simulink model "no_control1"  (R2018a)
settings: Solver=FixedStepAuto  StartTime=0.0  StopTime=50  FixedStep=2e-3  RelTol=1.0e-4
model workspace (MAT data in the model file):
  x1 = Simulink.Parameter
  x1.DataType = 'auto'
  x1.Dimensions = [0 0]
settings Model: Creator=Jay  LastModifiedBy=Jay
settings SolverCC: MaxConsecutiveZCs=1  ExtrapolationOrder=2  InsertRTBMode=Always

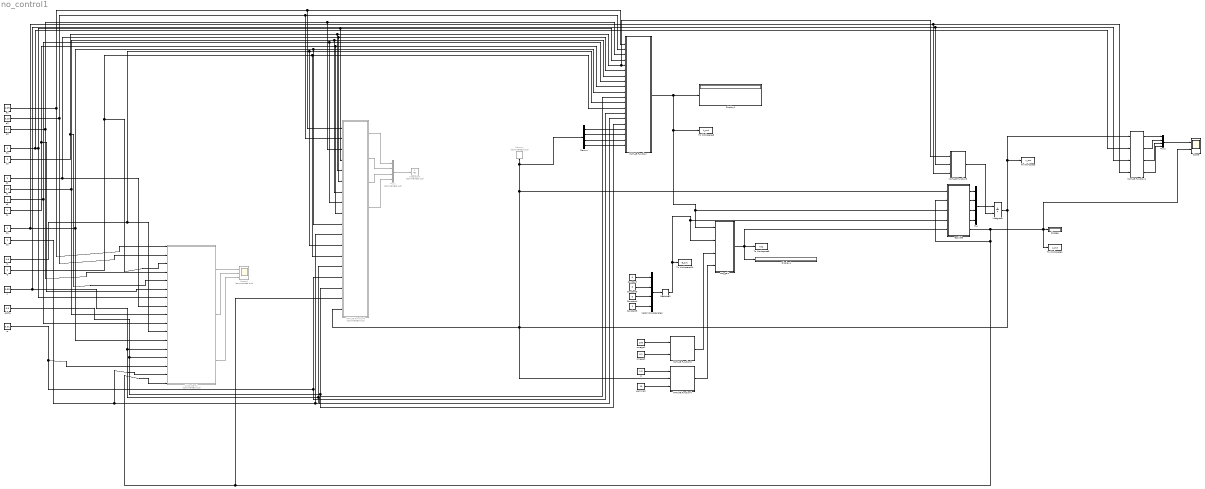
== system no_control1 ==
  Constant : Constant  Value=0
  Constant3 : Constant  Value=0
  Constant4 : Constant  Value=0
  Constant5 : Constant
  Demux : Demux
  Display1 : Display
  Display4 : Display
  Integrator : Integrator  InitialConditionSource=external  InitialCondition=[ 1-1; 0.2; 0.15-0.33/1; 0]
  Integrator2 : Integrator  Commented=on  InitialCondition=[1-1;0.2;0.15-0.33/0.2;0]
  MATLAB Function : MATLAB Function  TreatAsAtomicUnit=on
  MATLAB Function1 : MATLAB Function  TreatAsAtomicUnit=on
  MATLAB Function3 : MATLAB Function  TreatAsAtomicUnit=on
  MATLAB Function4 : MATLAB Function  TreatAsAtomicUnit=on
  MATLAB Function5 : MATLAB Function  TreatAsAtomicUnit=on
  MATLAB Function8 : MATLAB Function  Commented=on  TreatAsAtomicUnit=on
  Memory : Memory  Commented=on  InitialCondition=[0; 0.2; 0.15-0.33/1; 0]  InheritSampleTime=on
  Mux : Mux
  Mux1 : Mux  Commented=on
  Mux2 : Mux
  Reshape2 : Reshape  OutputDimensionality=Column vector (2-D)
  Scope : Scope  NumInputPorts=2
  Scope1 : Scope  Commented=on  NumInputPorts=3
  Subsystem1 : Subsystem  Commented=on
  To Workspace : ToWorkspace  VariableName=x_out  SaveFormat=Timeseries  SampleTime=-1
  To Workspace1 : ToWorkspace  VariableName=u_out  SaveFormat=Timeseries  SampleTime=-1
  To Workspace10 : ToWorkspace  VariableName=B_out  SaveFormat=Timeseries  SampleTime=-1
  To Workspace8 : ToWorkspace  VariableName=A_out  SaveFormat=Timeseries  SampleTime=-1
  To Workspace9 : ToWorkspace  VariableName=Kop  SaveFormat=Timeseries  SampleTime=-1
  Vector Concatenate2 : Concatenate  NumInputs=4  ConcatenateDimension=4
  a1 : Constant  Value=0.05
  a2 : Constant  Value=0.15
  a3 : Constant  Value=0.1
  alpha : Constant  Value=0.3
  are_gain : MATLAB Function  TreatAsAtomicUnit=on
  b1 : Constant
  b2 : Constant
  c1 : Constant
  c2 : Constant  Value=0.5
  c3 : Constant
  c4 : Constant
  d1 : Constant
  d2 : Constant
  dosage : Display
  gamma0 : Constant  Value=10
  omega1 : Constant  Value=100
  omega2 : Constant  Value=0.1
  r1 : Constant  Value=1.5
  r2 : Constant
  rc : Constant  Value=1.2
  regulate : MATLAB Function  TreatAsAtomicUnit=on
  ro : Constant  Value=0.01
  s : Constant  Value=0.33
  wires:
  regulate/5(u) -> regulate/2("u "), Subsystem1/17(u), MATLAB Function8/17(u), To Workspace1/1, dosage/1, Scope/2  "u"
  are_gain/1(Kop) -> regulate/5(Kop), To Workspace9/1, Display4/1
  MATLAB Function4/1(R) -> are_gain/4(R)  "R"
  MATLAB Function3/1(Q) -> are_gain/3(Q)  "Q"
  d2/1 -> Subsystem1/16(d2), MATLAB Function/11(d2), MATLAB Function8/11(d2)  "d2"
  omega1/1 -> MATLAB Function3/1(omega1)
  ro/1 -> MATLAB Function/14(ro), MATLAB Function8/15(ro), Subsystem1/15(ro)  "ro"
  c1/1 -> Subsystem1/8(c1), MATLAB Function8/6(c1), MATLAB Function/6(c1)  "c1"
  Reshape2/1 -> are_gain/2(B), regulate/4(B), To Workspace10/1  "B"
  Constant3/1 -> Vector Concatenate2/2
  gamma0/1 -> MATLAB Function4/3(gamma0)
  b1/1 -> MATLAB Function1/2(b1), Subsystem1/7(b1), MATLAB Function8/4(b1), MATLAB Function/4(b1)  "b1"
  alpha/1 -> MATLAB Function/16(alpha), MATLAB Function8/16(alpha), Subsystem1/14(alpha)  "alpha"
  d1/1 -> MATLAB Function1/4(d1), MATLAB Function5/3(d1), Subsystem1/12(d1), MATLAB Function/10(d1), MATLAB Function8/10(d1)  "d1"
  Constant4/1 -> Vector Concatenate2/3
  r1/1 -> Subsystem1/11(r1), MATLAB Function/12(r1), MATLAB Function8/12(r1)  "r1"
  a2/1 -> Subsystem1/2(a2), MATLAB Function/2(a2), MATLAB Function8/2(a2)  "a2"
  a3/1 -> Subsystem1/4(a3), MATLAB Function/3(a3), MATLAB Function8/3(a3)  "a3"
  c4/1 -> Subsystem1/6(c4), MATLAB Function8/9(c4), MATLAB Function/9(c4)  "c4"
  b2/1 -> Subsystem1/5(b2), MATLAB Function8/5(b2), MATLAB Function/5(b2), MATLAB Function5/1(b2)  "b2"
  Vector Concatenate2/1 -> Reshape2/1
  rc/1 -> MATLAB Function4/1(rc)
  Constant/1 -> Vector Concatenate2/1
  omega2/1 -> MATLAB Function3/2(omega2)
  MATLAB Function/1(A) -> regulate/3(A), are_gain/1(A), To Workspace8/1, Display1/1  "A"
  c2/1 -> Subsystem1/9(c2), MATLAB Function8/7(c2), MATLAB Function/7(c2)  "c2"
  r2/1 -> Subsystem1/3(r2), MATLAB Function/13(r2), MATLAB Function8/13(r2)  "r2"
  c3/1 -> Subsystem1/10(c3), MATLAB Function/8(c3), MATLAB Function8/8(c3)  "c3"
  a1/1 -> Subsystem1/1(a1), MATLAB Function/1(a1), MATLAB Function8/1(a1)  "a1"
  s/1 -> MATLAB Function/15(s), MATLAB Function8/14(s), Subsystem1/13(s), MATLAB Function1/3(s), MATLAB Function5/2(s)  "s"
  Integrator/1 -> MATLAB Function1/1(x), To Workspace/1, MATLAB Function4/2(x), Demux/1, Memory/1, regulate/1(x), MATLAB Function8/18(x)  "x"
  MATLAB Function8/1(x1_dot) -> Mux1/1
  MATLAB Function8/2(x2_dot) -> Mux1/2
  MATLAB Function8/3(x3_dot) -> Mux1/3
  MATLAB Function1/1(N) -> Mux2/1  "N"
  MATLAB Function1/2(T) -> Mux2/2  "T"
  MATLAB Function1/3(I) -> Mux2/3  "I"
  MATLAB Function1/4(M) -> Mux2/4  "M"
  Mux/1 -> Integrator/1
  regulate/1(x_dot1) -> Mux/1
  regulate/2(x_dot2) -> Mux/2
  regulate/3(x_dot3) -> Mux/3
  regulate/4(x_dot4) -> Mux/4
  Mux2/1 -> Scope/1
  Demux/1 -> MATLAB Function/17(x1)
  Demux/2 -> MATLAB Function/18(x2)
  Demux/3 -> MATLAB Function/19(x3)
  Demux/4 -> MATLAB Function/20(x4)
  MATLAB Function8/4(x4_dot) -> Mux1/4
  Mux1/1 -> Integrator2/1
  Subsystem1/3(Out3) -> Scope1/3
  Subsystem1/2(Out2) -> Scope1/2
  Subsystem1/1(Out1) -> Scope1/1
  Constant5/1 -> Vector Concatenate2/4
  MATLAB Function5/1(x_0) -> Integrator/2

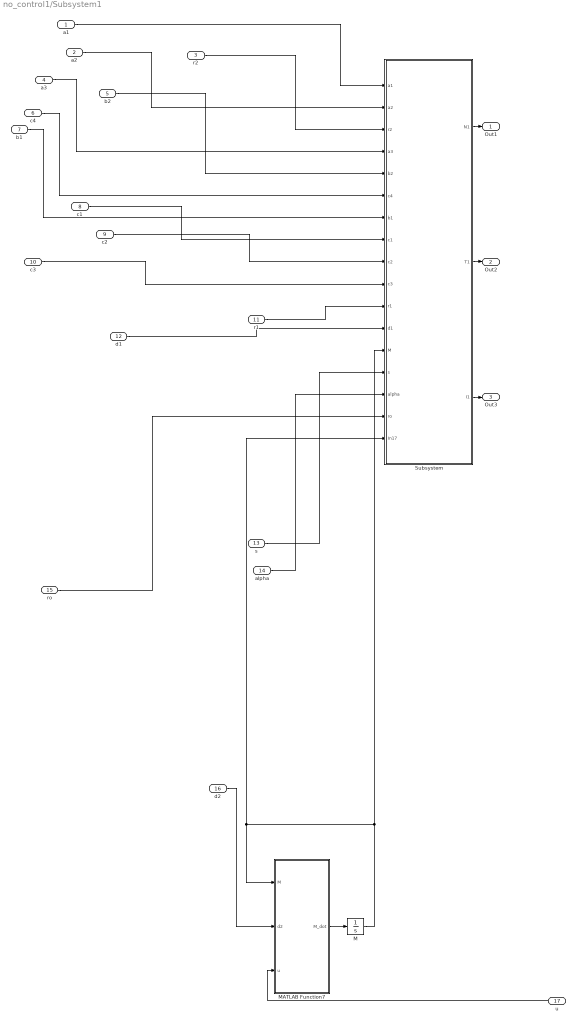
== system no_control1/Subsystem1 ==
  a1 : Inport
  a2 : Inport  Port=2
  r2 : Inport  Port=3
  a3 : Inport  Port=4
  b2 : Inport  Port=5
  c4 : Inport  Port=6
  b1 : Inport  Port=7
  c1 : Inport  Port=8
  c2 : Inport  Port=9
  c3 : Inport  Port=10
  r1 : Inport  Port=11
  d1 : Inport  Port=12
  s : Inport  Port=13
  alpha : Inport  Port=14
  ro : Inport  Port=15
  d2 : Inport  Port=16
  u : Inport  Port=17
  M : Integrator
  MATLAB Function7 : MATLAB Function  TreatAsAtomicUnit=on
  Subsystem : Subsystem
  Out1 : Outport
  Out2 : Outport  Port=2
  Out3 : Outport  Port=3
  wires:
  MATLAB Function7/1(M_dot) -> M/1
  Subsystem/1(N1) -> Out1/1
  Subsystem/3(I1) -> Out3/1
  r2/1 -> Subsystem/3(r2)
  M/1 -> Subsystem/13(M), Subsystem/17(In17), MATLAB Function7/1(M)
  r1/1 -> Subsystem/11(r1)
  c2/1 -> Subsystem/9(c2)
  u/1 -> MATLAB Function7/3(u)
  alpha/1 -> Subsystem/15(alpha)
  Subsystem/2(T1) -> Out2/1
  b1/1 -> Subsystem/7(b1)
  c1/1 -> Subsystem/8(c1)
  c3/1 -> Subsystem/10(c3)
  a1/1 -> Subsystem/1(a1)
  d1/1 -> Subsystem/12(d1)
  s/1 -> Subsystem/14(s)
  b2/1 -> Subsystem/5(b2)
  a3/1 -> Subsystem/4(a3)
  d2/1 -> MATLAB Function7/2(d2)
  c4/1 -> Subsystem/6(c4)
  a2/1 -> Subsystem/2(a2)
  ro/1 -> Subsystem/16(ro)

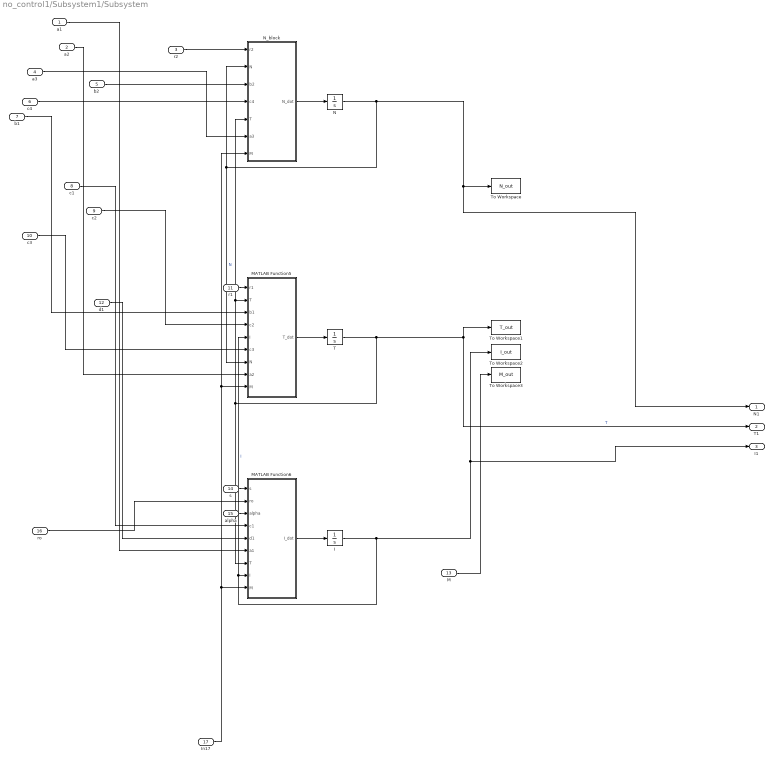
== system no_control1/Subsystem1/Subsystem ==
  a1 : Inport
  a2 : Inport  Port=2
  r2 : Inport  Port=3
  a3 : Inport  Port=4
  b2 : Inport  Port=5
  c4 : Inport  Port=6
  b1 : Inport  Port=7
  c1 : Inport  Port=8
  c2 : Inport  Port=9
  c3 : Inport  Port=10
  r1 : Inport  Port=11
  d1 : Inport  Port=12
  M : Inport  Port=13
  s : Inport  Port=14
  alpha : Inport  Port=15
  ro : Inport  Port=16
  In17 : Inport  Port=17
  I : Integrator  InitialCondition=0.15
  MATLAB Function5 : MATLAB Function  TreatAsAtomicUnit=on
  MATLAB Function6 : MATLAB Function  TreatAsAtomicUnit=on
  N : Integrator  InitialCondition=1
  N_block : MATLAB Function  TreatAsAtomicUnit=on
  T : Integrator  InitialCondition=0.25
  To Workspace : ToWorkspace  VariableName=N_out  SaveFormat=Timeseries  SampleTime=-1
  To Workspace1 : ToWorkspace  VariableName=T_out  SaveFormat=Timeseries  SampleTime=-1
  To Workspace2 : ToWorkspace  VariableName=I_out  SaveFormat=Timeseries  SampleTime=-1
  To Workspace3 : ToWorkspace  VariableName=M_out  SaveFormat=Timeseries  SampleTime=-1
  N1 : Outport
  T1 : Outport  Port=2
  I1 : Outport  Port=3
  wires:
  c4/1 -> N_block/4(c4)
  c2/1 -> MATLAB Function5/4(c2)
  N/1 -> MATLAB Function5/7(N), N_block/2(N), N1/1, To Workspace/1  "N"
  In17/1 -> N_block/7(M), MATLAB Function5/9(M), MATLAB Function6/9(M)
  a1/1 -> MATLAB Function6/6(a1)
  N_block/1(N_dot) -> N/1
  I/1 -> I1/1, To Workspace2/1, MATLAB Function5/5(I), MATLAB Function6/8(I)  "I"
  T/1 -> MATLAB Function6/7(T), N_block/5(T), MATLAB Function5/2(T), T1/1, To Workspace1/1  "T"
  MATLAB Function6/1(I_dot) -> I/1
  M/1 -> To Workspace3/1
  b1/1 -> MATLAB Function5/3(b1)
  MATLAB Function5/1(T_dot) -> T/1
  s/1 -> MATLAB Function6/1(s)
  c3/1 -> MATLAB Function5/6(c3)
  alpha/1 -> MATLAB Function6/3(alpha)
  d1/1 -> MATLAB Function6/5(d1)
  r2/1 -> N_block/1(r2)
  b2/1 -> N_block/3(b2)
  ro/1 -> MATLAB Function6/2(ro)
  a3/1 -> N_block/6(a3)
  a2/1 -> MATLAB Function5/8(a2)
  c1/1 -> MATLAB Function6/4(c1)
  r1/1 -> MATLAB Function5/1(r1)

== matlab function no_control1/MATLAB Function1 ==
  data: x input; N output; b1 input; T output; I output; M output; s input; d1 input
function [N,T,I,M] = fcn(x,b1,s,d1)
    
    N = x(1) + 1/b1;
    T = x(2);
    I = x(3) + s/d1;
    M = x(4);

== matlab function no_control1/MATLAB Function ==
  data: a1 input; a2 input; a3 input; b1 input; b2 input; c1 input; c2 input; c3 input; c4 input; d1 input; d2 input; r1 input; r2 input; ro input; A output; s input; alpha input; x1 input; x2 input; x3 input; x4 input
function A =  f_A(a1,a2,a3,b1,b2,c1,c2,c3,c4,d1,d2,r1,r2,ro,s,alpha,x1,x2,x3,x4)

    A11 =  -r2*(1+b2*x1);
    A12 =  -c4*(x1 + 1/b2);
    A13 =  0;
    A14 =  -a3*(1/b2 + x1);

    A21 =  -c3*x2;
    A22 =  r1*(1-b1*x2)-(c2*s/d1 + c3/b2);
    A23 =  -c2*x2;
    A24 =  -a2*x2;

    A31 =  0;
%     A32 =  -(s + d1*x3)*(alpha*c1 - ro + c1*x2)/(d1*(alpha + x2)); % new
    A32 = ro*(x3 + s/d1)/(alpha + x2) -c1*(x3+s/d1) -x4; % default
    A33 =  -d1;
%     A34 =  -(a1*(s + d1*x3))/d1; % new
    A34 =  -a1*(x3 + s/d1)+x2; % default
    
    A41 =  0;
    A42 =  0;
    A43 =  0;
    A44 =  -d2; %%% *x4
   
    
    A = [  A11 A12 A13 A14;% -1.0000   -1.0000         0   -0.1000;
           A21 A22 A23 A24;% -0.2000   -0.6250   -0.1000   -0.0300;
           A31 A32 A33 A34;
           %0   -0.1470   -0.2000    0.1925;
           A41 A42 A43 A44];%      0         0         0   -1.0000];
           
%    -0.0400   -0.2795   -0.0375
%    -0.9603   -1.0000    0.0190
%     0.0000    0.0000   -1.0000

%     x_dot1 = -r2*x1*(1 +b2*x1) -c4/b2*x2 -a3/b2*x4 -c4*x1*x2 -a3*x1*x4;  
%     x_dot2 = r1*x2*(1-b1*x2) -(c2*s/d1 + c3/b2)*x2 -c3*x1*x2 -c2*x2*x3 -a2*x2*x4;
%     x_dot3 = -c2*s/d1*x2 -d1*x3 -a1*s/d1*x4 +(ro*s/d1)*x2/(alpha+x2) +ro*x2*x3/(alpha+x2) -c1*x2*x3 -a1*x3*x4;
% % % %     x_dot33 = -x2*(s + d1*x3)*(alpha*c1 - ro + c1*x2)/(d1*(alpha + x2)) - d1*x3 - x4*(a1*(s + d1*x3))/d1;
%     x_dot4 = -d2*x4;% +u;
%     
%     x_dot = [x_dot1; x_dot2; x_dot3; x_dot4];

== matlab function no_control1/Subsystem1/Subsystem/N_block ==
  data: r2 input; N_dot output; N input; b2 input; c4 input; T input; a3 input; M input
function N_dot = fcn(r2,N,b2,c4,T,a3,M)
    
    N_dot = r2*N*(1-b2*N)-c4*T*N-a3*M*N;

== matlab function no_control1/MATLAB Function3 ==
  data: Q output; omega1 input; omega2 input
function Q = f_Q(omega1, omega2)
    Q = [ 0 0 0 0; 0 omega1 0 0; 0 0 0 0; 0 0 0 omega2];

== matlab function no_control1/MATLAB Function4 ==
  data: R output; rc input; x input; gamma0 input
function R = f_R(rc,x,gamma0)
    
    x2 = x(2);
    R = rc;
%     R = rc +gamma0*x2;

== matlab function no_control1/Subsystem1/Subsystem/MATLAB Function5 ==
  data: r1 input; T input; b1 input; c2 input; I input; c3 input; T_dot output; N input; a2 input; M input
function T_dot = fcn(r1,T,b1,c2,I,c3,N,a2,M)
    
    T_dot = r1*T*(1-b1*T)-c2*I*T-c3*T*N-a2*M*T;

== matlab function no_control1/Subsystem1/Subsystem/MATLAB Function6 ==
  data: s input; ro input; alpha input; c1 input; d1 input; a1 input; T input; I input; I_dot output; M input
function I_dot = fcn(s,ro,alpha,c1,d1,a1,T,I,M)
    
    I_dot = s + ro*I*T/(alpha+T) - c1*I*T - d1*I - a1*M*I;

== matlab function no_control1/Subsystem1/MATLAB Function7 ==
  data: M input; d2 input; u input; M_dot output
function M_dot = fcn(M,d2,u)
%     u=0;
%     M_dot = -d2*M - u;
    M_dot = 0;

== matlab function no_control1/MATLAB Function8 ==
  data: a1 input; a2 input; a3 input; b1 input; b2 input; c1 input; c2 input; c3 input; c4 input; d1 input; d2 input; r1 input; r2 input; x1_dot output; s input; ro input; alpha input; u input; x2_dot output; x3_dot output; x4_dot output; x input; x1 output; x2 output; x3 output; x4 output
function [x1_dot, x2_dot, x3_dot, x4_dot, x1, x2, x3, x4] = fcn(a1, a2, a3, b1, b2, c1, c2, c3, c4, d1, d2, r1, r2, s, ro, alpha, u, x)
    
%     x1 = N-1/b2;
%     x2 = T;
%     x3 = I-s/d1;
%     x4 = M;
%%%%%%%%%%%%%%%%%%%%%%%%%%%%%%
    x1 = x(1);
    x2 = x(2);
    x3 = x(3);
    x4 = x(4);
    
    x1_dot = -r2*x1*(1 +b2*x1) -c4/b2*x2 -a3/b2*x4 -c4*x1*x2 -a3*x1*x4;  
    x2_dot = r1*x2*(1-b1*x2) -(c2*s/d1 + c3/b2)*x2 -c3*x1*x2 -c2*x2*x3 -a2*x2*x4;
    x3_dot = -c2*s/d1*x2 -d1*x3 -a1*s/d1*x4 +(ro*s/d1)*x2/(alpha+x2) +ro*x2*x3/(alpha+x2) -c1*x2*x3 -a1*x3*x4;
    x4_dot = -d2*x4 +u;

== matlab function no_control1/regulate ==
  data: x input; u input; A input; B input; x_dot1 output; x_dot2 output; x_dot3 output; x_dot4 output; u output; Kop input
function [x_dot1,x_dot2,x_dot3,x_dot4,u] = regulate(x,u,A,B,Kop)
        
    x_dot1 = 0;
    x_dot2 = 0;
    x_dot3 = 0;
    x_dot4 = 0;
    
    u_min=0;
    u_max=1;
    
    u_unb = 0;
    u_bound = 0;
    u=0;

%     x_dot = [-100;-100;-100;-100];
%     A-(B*Kop)
    
    x_dot = (A-B*Kop)*x; % Closed loop system
%   must be  x_dot = A*x+B*u;
    
%     x_dot1 = x_dot(1);
%     x_dot2 = x_dot(2);
%     x_dot3 = x_dot(3);
%     x_dot4 = x_dot(4);
%     [-Kop(1)*x(1)     -Kop(2)*x(2)     -Kop(3)*x(3)     -Kop(4)*x(4)]
    
    u_unb = -Kop*x;
    u_bound = min(max(u_unb,u_min),u_max);
    
    u = u_unb; 
%     u = u_bound;
%     u = 0;

    x_dot1 = x_dot(1);
    x_dot2 = x_dot(2);
    x_dot3 = x_dot(3);
    x_dot4 = x_dot(4);
    
%     x_dot1 = x(1);
%     x_dot2 = x(2);
%     x_dot3 = x(3);
%     x_dot4 = x(4);

== matlab function no_control1/are_gain ==
  data: A input; Kop output; B input; Q input; R input
function Kop = are_gain(A,B,Q,R)
    
coder.extrinsic('lqr','care','dare','are','ordschur','mat2cell');

% Initialise
Kop = [1 1 1 1];

% Ad = A(1).data;
% Bd = B.data;
% A = [-2 -2 0 -0.2; -0.2 -0.625 -0.1 -0.3; 0 -1.764 -0.2 0.11; 0 0 0 -1];
% B = [0;0;0;1];
% Q = [0 0 0 0; 0 100.0000 0 0; 0 0 0 0; 0 0 0 0.1000];
% R = 1;

% [Kop,~,~] = lqr(A,B,Q,R);
 
% P = ARE_diag(A,B,Q,R);

% Kop = [0 0 0 0];
%%
% P = Riccati(A,B,Q,R);

[P,K,L] = dare(A,B,Q,R);

% [P,K,L] = care(A,B,Q,R);

Kop = (R^-1)*(B')*P;


%%

% H = [A, -B/R*B'; -Q, -A'];
% 
% [U, S] = schur(H);
% 
% [U, S] = ordschur(U, S, 'lhp');
% 
% [m,n] = size(U);
% U11 = U(1:(m/2), 1:(n/2));
% U21 = U((m/2+1):m, 1:(n/2));
% 
% X = U21/U11;
% 
% Kop = (R^-1)*(B')*X;

== matlab function no_control1/MATLAB Function5 ==
  data: x_0 output; b2 input; s input; d1 input
function x_0 = init_x(b2,s,d1)

    N_0 = 1; T_0 = 0.2; I_0 = 0.15; M_0 = 0;
    
    x1_0 = N_0 - 1/b2;
    x2_0 = T_0;
    x3_0 = I_0 - s/d1;
    x4_0 = M_0;
    
    x_0 = [x1_0; x2_0; x3_0; x4_0];
